simulink model "AFEsimple"  (R2013b)
settings: Solver=FixedStepDiscrete  StartTime=0.0  StopTime=0.2  FixedStep=Tpas  RelTol=1e-3
InitFcn:
  | Ts = 1e-5
values from neighbouring files (symbols this model uses):
  Freq = 50    [AFE_2L_RC_param_DT1.m]    (also in AFE_FV_Params.m; AFE_PontHPV2.m; AFEsimplepara.m; AFEsimpleparaDT1.m)
  Iac = 2000    [AFEsimplepara.m]
  Lac = 8.1487e-04    (= 0.00081487)    [AFE_2L_RC_param_DT1.m]    (also in AFE_FV_Params.m; AFE_PontHPV2.m; AFEsimplepara.m = 0.002; AFEsimpleparaDT1.m)
  Phase = 300    [AFEsimplepara.m]
  Rac = 2.5    [AFEsimplepara.m]
  Tpas = 5e-5    (= 5e-05)    [AFE_2L_RC_param_DT1.m]    (also in AFE_FV_Params.m; AFE_PontHPV2.m = 3e-06; AFEsimplepara.m = 1e-05; AFEsimpleparaDT1.m)
  Vac = 2000    [AFE_2L_RC_param_DT1.m]    (also in AFE_FV_Params.m; AFE_PontHPV2.m; AFEsimplepara.m; AFEsimpleparaDT1.m)
libraries: powerlib x32, powerlib_extras x3, powerlib_meascontrol x1
settings Model: Creator=LiberT  LastModifiedBy=LiberT
settings DataIOCC: SignalLoggingSaveFormat=ModelDataLogs
settings OptimizationCC: ExpressionDepthLimit=2147483647
settings DebuggingCC: FcnCallInpInsideContextMsg=EnableAllAsWarning  StateNameClashWarn=warning

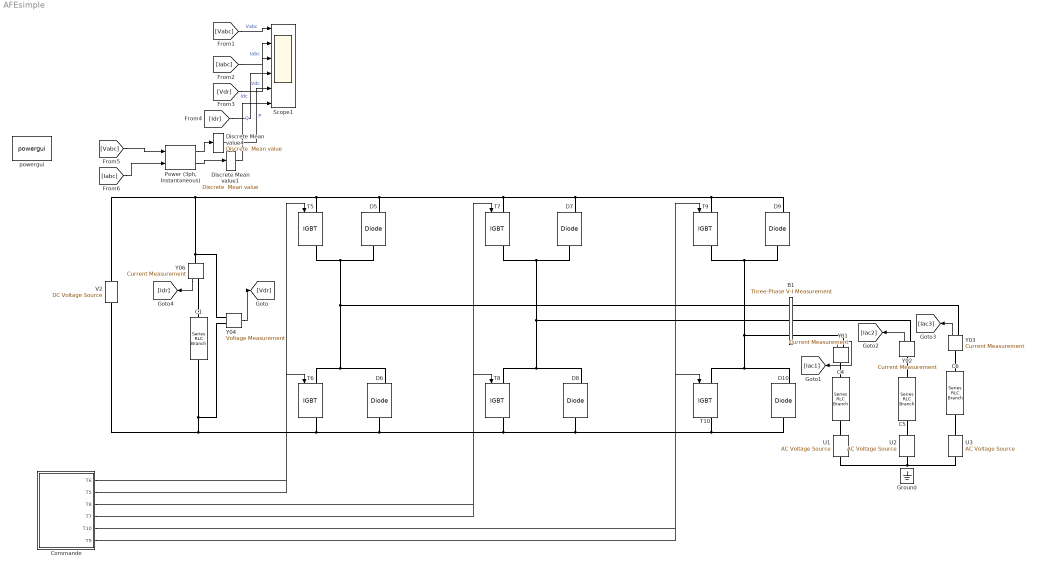
== system AFEsimple ==
  B1 : powerlib/Measurements/Three-Phase V-I Measurement  VoltageMeasurement=phase-to-phase  SetLabelV=on  LabelV=Vabc  Vpu=off  VpuLL=off  CurrentMeasurement=yes  SetLabelI=on  LabelI=Iabc  Ipu=off  Pbase=100e6  Vbase=500e3  OutputType=Complex  PhasorSimulation=off  PSBequivalent=0
  C1 : powerlib/Elements/Series RLC Branch  LConnTagsString=__new0  RConnTagsString=__new0  BranchType=R  Resistance=Rac  Inductance=Lac  SetiL0=off  InitialCurrent=0  Capacitance=300e-3  Setx0=off  InitialVoltage=0  Measurements=None
  C4 : powerlib/Elements/Series RLC Branch  LConnTagsString=__new0  RConnTagsString=__new0  BranchType=L  Resistance=Rac  Inductance=Lac  SetiL0=off  InitialCurrent=0  Capacitance=300e-3  Setx0=off  InitialVoltage=0  Measurements=None
  C5 : powerlib/Elements/Series RLC Branch  LConnTagsString=__new0  RConnTagsString=__new0  BranchType=L  Resistance=Rac  Inductance=Lac  SetiL0=off  InitialCurrent=0  Capacitance=300e-3  Setx0=off  InitialVoltage=0  Measurements=None
  C6 : powerlib/Elements/Series RLC Branch  LConnTagsString=__new0  RConnTagsString=__new0  BranchType=L  Resistance=Rac  Inductance=Lac  SetiL0=off  InitialCurrent=0  Capacitance=300e-3  Setx0=off  InitialVoltage=0  Measurements=None
  Commande : Subsystem
  D{5..10} (6 alike) : powerlib/Power Electronics/Diode  Ron=0.001  Lon=0  Vf=0.8  IC=0  UseSnubber=off  Rs=500  Cs=250e-9  Measurements=on
  Discrete Mean value1 : powerlib_extras/Discrete Measurements/Discrete  Mean value  Freq=Freq  Vinit=0  Ts=Tpas
  Discrete Mean value4 : powerlib_extras/Discrete Measurements/Discrete  Mean value  Freq=Freq  Vinit=0  Ts=Tpas
  Ground : powerlib/Elements/Ground  LConnTagsString=a
  "Power (3ph, Instantaneous)" : powerlib_meascontrol/Measurements/Power (3ph, Instantaneous)
  Scope1 : Scope  NumInputPorts=6
      settings: TickLabels=on  TimeRange=0.2  YMin=-7500~-3000~4750~1900~-3.5e+06~-5e+06  YMax=7500~3000~5250~2100~-3e+06~-4.65e+06
  T{5..10} (6 alike) : powerlib/Power Electronics/IGBT  Ron=0.001  Lon=0  Vf=1  Tf=1e-6  Tt=2e-6  IC=0  Rs=1e5  Cs=inf  Measurements=on
  U1 : powerlib/Electrical Sources/AC Voltage Source  Amplitude=Vac  Phase=0  Frequency=Freq  SampleTime=0  Measurements=None
  U2 : powerlib/Electrical Sources/AC Voltage Source  Amplitude=Vac  Phase=120  Frequency=Freq  SampleTime=0  Measurements=None
  U3 : powerlib/Electrical Sources/AC Voltage Source  Amplitude=Vac  Phase=240  Frequency=Freq  SampleTime=0  Measurements=None
  V2 : powerlib/Electrical Sources/DC Voltage Source  Amplitude=5000  Measurements=None
  Y01 : powerlib/Measurements/Current Measurement  PhasorSimulation=off  OutputType=Complex  PSBequivalent=0
  Y02 : powerlib/Measurements/Current Measurement  PhasorSimulation=off  OutputType=Complex  PSBequivalent=0
  Y03 : powerlib/Measurements/Current Measurement  PhasorSimulation=off  OutputType=Complex  PSBequivalent=0
  Y04 : powerlib/Measurements/Voltage Measurement  PhasorSimulation=off  OutputType=Complex  PSBequivalent=0
  Y06 : powerlib/Measurements/Current Measurement  PhasorSimulation=off  OutputType=Complex  PSBequivalent=0
  powergui : powerlib/powergui  Priority=1  SimulationMode=Discrete  SolverType=Tustin  SampleTime=Tpas  frequency=60  SPID=off  DisableSnubberDevices=off  DisableRonSwitches=off  DisableVfSwitches=off  SwTol=0  Interpol=off  DisplayEquations=off  frequencyindice=0  Pbase=100e6  ErrMax=1e-4  Iterations=50  UnitsV=kV  UnitsW=MW  FunctionMessages=off  echomessages=off  HookPort=off  EnableUseOfTLC=off  x0status=blocks  RestoreLinks=warning  ResistiveCurrentMeasurement=off  Frange=[0:2:500]  Ylog=off  Xlog=on  ShowGrid=off  save=off  variable=ZData  ZoomFFT=off  StartTime=0.0  cycles=1  DisplayStyle=1  fundamental=60  FreqAxis=off  MaxFrequency=1000  frequencyindicesteady=1  RmsSteady=1  display=off  Ts=0  methode=off
  wires:
  Y04/1 -> [Vdr]
  Commande/6(T9) -> T9/1
  Commande/5(T10) -> T10/1
  Commande/4(T7) -> T7/1
  Commande/3(T8) -> T8/1
  [Vabc] -> Scope1/1  "Vabc"
  [Iabc] -> Scope1/2  "Iabc"
  Commande/2(T5) -> T5/1
  Commande/1(T6) -> T6/1
  Y01/1 -> [Iac1]
  Y02/1 -> [Iac2]
  Y03/1 -> [Iac3]
  [Vdr] -> Scope1/3  "Vdc"
  [Idr] -> Scope1/4  "Idc"
  "Power (3ph, Instantaneous)"/1 -> Discrete Mean value4/1
  "Power (3ph, Instantaneous)"/2 -> Discrete Mean value1/1
  Discrete Mean value4/1 -> Scope1/5  "P"
  Discrete Mean value1/1 -> Scope1/6  "Q"
  [Vabc] -> "Power (3ph, Instantaneous)"/1
  [Iabc] -> "Power (3ph, Instantaneous)"/2
  Y06/1 -> [Idr]
  connections:
  T6/RConn1 -- V2/LConn1 -- C1/RConn1 -- Y04/LConn2 -- T8/RConn1 -- D8/LConn1 -- T10/RConn1 -- D10/LConn1 -- D6/LConn1
  T9/RConn1 -- D9/LConn1 -- T10/LConn1 -- D10/RConn1 -- B1/LConn3
  T5/LConn1 -- V2/RConn1 -- Y04/LConn1 -- Y06/LConn1 -- D5/RConn1 -- D7/RConn1 -- T9/LConn1 -- D9/RConn1 -- T7/LConn1
  T8/LConn1 -- D8/RConn1 -- T7/RConn1 -- D7/LConn1 -- B1/LConn2
  T5/RConn1 -- D5/LConn1 -- T6/LConn1 -- D6/RConn1 -- B1/LConn1
  U1/RConn1 -- C4/RConn1
  U2/RConn1 -- C5/RConn1
  U3/RConn1 -- C6/RConn1
  U1/LConn1 -- U3/LConn1 -- U2/LConn1
  C4/LConn1 -- Y01/LConn1
  Y01/RConn1 -- B1/RConn3
  C5/LConn1 -- Y02/LConn1
  Y02/RConn1 -- B1/RConn2
  Y03/LConn1 -- C6/LConn1
  Y03/RConn1 -- B1/RConn1
  Y06/RConn1 -- C1/LConn1

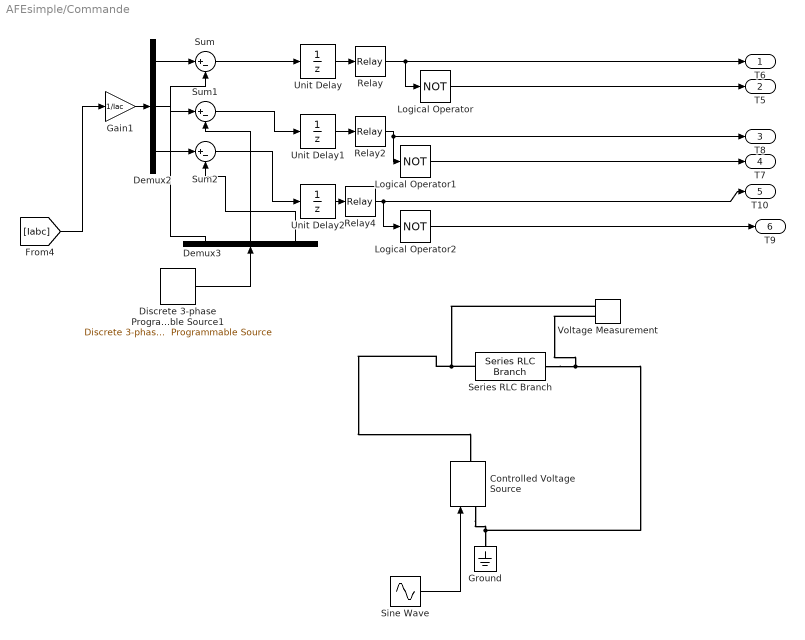
== system AFEsimple/Commande ==
  Controlled Voltage Source : powerlib/Electrical Sources/Controlled Voltage Source  Initialize=on  Source_Type=AC  Amplitude=2000  Phase=0  Frequency=0  Measurements=None
  Demux2 : Demux  Outputs=3
  Demux3 : Demux  Outputs=3
  Discrete 3-phase Programmable Source1 : powerlib_extras/Discrete  Control Blocks/Discrete 3-phase  Programmable Source  Par_Vps=[Iac/Iac Phase Freq]  VariationEntity=None  VariationType=Step  VariationStep=-0.5  VariationRate=10  VariationMag=0.3  VariationFreq=2  Par_Timing_Variation=[0.1 1.2]  SinglePhase=on  Yampli=[1 0.2 1.2 1.0]  Xtime=[0 0.1 0.15 0.2]  HarmonicGeneration=off  Par_HarmoA=[3 0.2 -25 0]  Par_HarmoB=[2 0.15 35 2]  Par_Timing_Harmo="[0.05  3]"  Ts=Tpas
  Gain1 : Gain  Gain=1/Iac
  Ground : powerlib/Elements/Ground  LConnTagsString=a
  Logical Operator : Logic  Operator=NOT  AllPortsSameDT=off
  Logical Operator1 : Logic  Operator=NOT  AllPortsSameDT=off
  Logical Operator2 : Logic  Operator=NOT  AllPortsSameDT=off
  Relay : Relay  OnSwitchValue=0.05  OffSwitchValue=-0.05
  Relay2 : Relay  OnSwitchValue=0.05  OffSwitchValue=-0.05
  Relay4 : Relay  OnSwitchValue=0.05  OffSwitchValue=-0.05
  Series RLC Branch : powerlib/Elements/Series RLC Branch  LConnTagsString=__new0  RConnTagsString=__new0  BranchType=R  Resistance=1000  Inductance=1e-3  SetiL0=off  InitialCurrent=0  Capacitance=1e-6  Setx0=off  InitialVoltage=0  Measurements=None
  Sine Wave : Sin  Amplitude=2000  Frequency=314.159  SampleTime=0
  Sum : Sum  Inputs=|+-
  Sum1 : Sum  Inputs=|+-
  Sum2 : Sum  Inputs=|+-
  Unit Delay : UnitDelay  SampleTime=-1
  Unit Delay1 : UnitDelay  SampleTime=-1
  Unit Delay2 : UnitDelay  SampleTime=-1
  Voltage Measurement : powerlib/Measurements/Voltage Measurement  PhasorSimulation=off  OutputType=Complex  PSBequivalent=0
  T6 : Outport
  T5 : Outport  Port=2
  T8 : Outport  Port=3
  T7 : Outport  Port=4
  T10 : Outport  Port=5
  T9 : Outport  Port=6
  wires:
  Demux2/1 -> Sum/1
  Demux3/1 -> Sum/2
  Demux2/2 -> Sum1/1
  Demux2/3 -> Sum2/1
  Demux3/2 -> Sum1/2
  Demux3/3 -> Sum2/2
  Gain1/1 -> Demux2/1
  Discrete 3-phase Programmable Source1/1 -> Demux3/1
  Relay/1 -> T6/1, Logical Operator/1
  Logical Operator/1 -> T5/1
  Relay2/1 -> T8/1, Logical Operator1/1
  Logical Operator1/1 -> T7/1
  Relay4/1 -> Logical Operator2/1, T10/1
  Logical Operator2/1 -> T9/1
  Sine Wave/1 -> Controlled Voltage Source/1
  Sum/1 -> Unit Delay/1
  Unit Delay/1 -> Relay/1
  Unit Delay1/1 -> Relay2/1
  Sum1/1 -> Unit Delay1/1
  Sum2/1 -> Unit Delay2/1
  Unit Delay2/1 -> Relay4/1
  [Iabc] -> Gain1/1
  connections:
  Controlled Voltage Source/LConn1 -- Voltage Measurement/LConn2 -- Series RLC Branch/RConn1 -- Ground/LConn1
  Series RLC Branch/LConn1 -- Voltage Measurement/LConn1 -- Controlled Voltage Source/RConn1
